simulink model "smart_sim"  (Simulink 8.0)
settings: Solver=ode45  StartTime=0.0  StopTime=256*2000  RelTol=1e-3
libraries: xbsIndex_r4 x75, simulink x1, xps_library x1
settings Model: Creator=kids  LastModifiedBy=kids

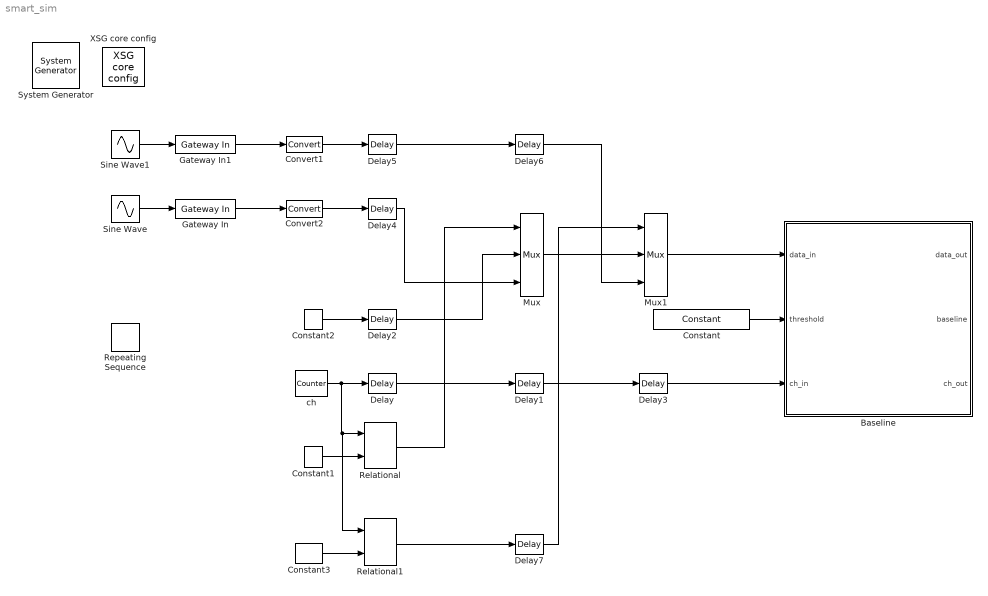
== system smart_sim ==
  " System Generator" : xbsIndex_r4/ System Generator  Tag=genX  xilinxfamily=virtex5  part=xc5vsx95t  speed=-1  package=ff1136  synthesis_tool=XST  clock_wrapper=Clock Enables  directory=./chan_dead_v1/sysgen  proj_type=Project Navigator  Synth_file=XST Defaults  Impl_file=ISE Defaults  testbench=off  simulink_period=1  sysclk_period=3.9062  dcm_input_clock_period=100  incr_netlist=off  trim_vbits=Everywhere in SubSystem  dbl_ovrd=According to Block Masks  core_generation=According to Block Masks  run_coregen=off  deprecated_control=off  eval_field=0  block_type=sysgen
      settings: block_version=10.1.3
  Baseline : Subsystem  mask{logChannels=8, logPtsInAvg=10, logSamplePeriod=1}
      mask prompts: logChannels "number of channels 2^M"; logPtsInAvg "number of samples per average 2^N"; logSamplePeriod "sampling period 2^P"
  Constant : xbsIndex_r4/Constant  const=-.1  gui_display_data_type=Fixed-point  arith_type=Signed (2's comp)  n_bits=16  bin_pt=13  preci_type=Single  exp_width=8  frac_width=24  explicit_period=off  period=1  equ=P=C  opselect=C  inp2=PCIN>>17  opr=+  inp1=P  carry=CIN  dbl_ovrd=off  block_type=constant
  Constant1 : xbsIndex_r4/Constant  const=1  gui_display_data_type=Fixed-point  arith_type=Signed (2's comp)  n_bits=4  bin_pt=0  preci_type=Single  exp_width=8  frac_width=24  explicit_period=off  period=1  equ=P=C  opselect=C  inp2=PCIN>>17  opr=+  inp1=P  carry=CIN  dbl_ovrd=off  block_type=constant
  Constant2 : xbsIndex_r4/Constant  const=0  gui_display_data_type=Fixed-point  arith_type=Signed (2's comp)  n_bits=16  bin_pt=13  preci_type=Single  exp_width=8  frac_width=24  explicit_period=on  period=1  equ=P=C  opselect=C  inp2=PCIN>>17  opr=+  inp1=P  carry=CIN  dbl_ovrd=off  block_type=constant
  Constant3 : xbsIndex_r4/Constant  const=10  gui_display_data_type=Fixed-point  arith_type=Unsigned  n_bits=4  bin_pt=0  preci_type=Single  exp_width=8  frac_width=24  explicit_period=off  period=1  equ=P=C  opselect=C  inp2=PCIN>>17  opr=+  inp1=P  carry=CIN  dbl_ovrd=off  block_type=constant
  Convert1 : xbsIndex_r4/Convert  gui_display_data_type=Fixed-point  arith_type="Signed  (2's comp)"  n_bits=16  bin_pt=13  float_type=Single  exp_bits=8  fraction_bits=24  quantization=Truncate  overflow=Wrap  en=off  latency=0  dbl_ovrd=off  pipeline=off  block_type=convert
      settings: block_version=11.4
  Convert2 : xbsIndex_r4/Convert  gui_display_data_type=Fixed-point  arith_type="Signed  (2's comp)"  n_bits=16  bin_pt=13  float_type=Single  exp_bits=8  fraction_bits=24  quantization=Truncate  overflow=Wrap  en=off  latency=0  dbl_ovrd=off  pipeline=off  block_type=convert
      settings: block_version=11.4
  Delay{,1..7} (8 alike) : xbsIndex_r4/Delay  rst=off  infoeditControl=Selection of Reset will increase slice count due to use of real FFs and instead of SRLs  en=off  latency=1  dbl_ovrd=off  reg_retiming=off  block_type=delay
  Gateway In : xbsIndex_r4/Gateway In  gui_display_data_type=Fixed-point  arith_type="Signed  (2's comp)"  n_bits=16  bin_pt=13  preci_type=Single  exp_width=8  frac_width=24  quantization="Round  (unbiased: +/- Inf)"  overflow=Saturate  period=1  dbl_ovrd=off  timing_constraint=None  locs_specified=off  LOCs={}  UseAsADC=off  ADCChannel='1'  inherit_from_input=off  hdl_port=on  block_type=gatewayin
  Gateway In1 : xbsIndex_r4/Gateway In  gui_display_data_type=Fixed-point  arith_type="Signed  (2's comp)"  n_bits=16  bin_pt=13  preci_type=Single  exp_width=8  frac_width=24  quantization="Round  (unbiased: +/- Inf)"  overflow=Saturate  period=1  dbl_ovrd=off  timing_constraint=None  locs_specified=off  LOCs={}  UseAsADC=off  ADCChannel='1'  inherit_from_input=off  hdl_port=on  block_type=gatewayin
  Mux : xbsIndex_r4/Mux  inputs=2  en=off  latency=1  precision=Full  arith_type=Unsigned  n_bits=16  bin_pt=14  quantization=Truncate  overflow=Wrap  dbl_ovrd=off  block_type=mux
  Mux1 : xbsIndex_r4/Mux  inputs=2  en=off  latency=1  precision=Full  arith_type=Unsigned  n_bits=16  bin_pt=14  quantization=Truncate  overflow=Wrap  dbl_ovrd=off  block_type=mux
  Relational : xbsIndex_r4/Relational  mode=a=b  en=off  latency=1  dbl_ovrd=off  block_type=relational
  Relational1 : xbsIndex_r4/Relational  mode=a=b  en=off  latency=1  dbl_ovrd=off  block_type=relational
  Repeating Sequence : simulink/Sources/Repeating Sequence  rep_seq_t=[0 16 16+1 2*16]  rep_seq_y=[1 1 2 2]
  Sine Wave : Sin  SineType=Sample based  Amplitude=.25  Bias=.75  Frequency=100  Samples=50*256  SampleTime=1
  Sine Wave1 : Sin  SineType=Sample based  Amplitude=.5  Bias=1.2  Frequency=100  Samples=20*256  SampleTime=1
  XSG core config : xps_library/XSG core config  Tag=xps:xsg  hw_sys=ROACH:sx95t  clk_src=adc1_clk  ROACH_clk_src=adc1_clk  ROACH2_clk_src=adc0_clk  clk_rate=256  sample_period=1  synthesis_tool=XST
  ch : xbsIndex_r4/Counter  cnt_type=Free Running  cnt_to=4  operation=Up  start_count=0  cnt_by_val=1  arith_type=Unsigned  n_bits=8  bin_pt=0  load_pin=off  rst=off  en=off  explicit_period=on  period=1  dbl_ovrd=off  use_behavioral_HDL=off  implementation=Fabric  block_type=counter
  wires:
  ch/1 -> Relational1/1, Relational/1, Delay/1
  Constant/1 -> Baseline/2(threshold)
  Constant1/1 -> Relational/2
  Constant2/1 -> Delay2/1
  Delay/1 -> Delay1/1
  Delay1/1 -> Delay3/1
  Delay2/1 -> Mux/2
  Convert2/1 -> Delay4/1
  Gateway In/1 -> Convert2/1
  Sine Wave/1 -> Gateway In/1
  Gateway In1/1 -> Convert1/1
  Sine Wave1/1 -> Gateway In1/1
  Constant3/1 -> Relational1/2
  Relational/1 -> Mux/1
  Mux/1 -> Mux1/2
  Relational1/1 -> Delay7/1
  Convert1/1 -> Delay5/1
  Mux1/1 -> Baseline/1(data_in)
  Delay3/1 -> Baseline/3(ch_in)
  Delay4/1 -> Mux/3
  Delay5/1 -> Delay6/1
  Delay6/1 -> Mux1/3
  Delay7/1 -> Mux1/1

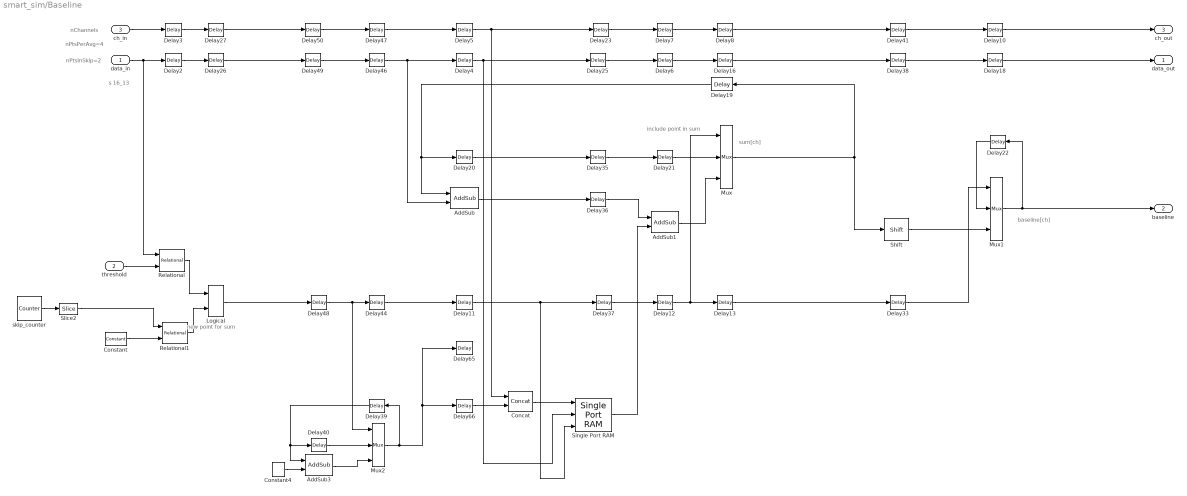
== system smart_sim/Baseline ==
  note: sum[ch]
  note: baseline[ch]
  note: nPtsInSkip=2
  note: nPtsPerAvg=4
  note: new point
      | for sum
  note: nChannels
  note: include point in sum
  note: s 16_13
  data_in : Inport
  threshold : Inport  Port=2
  ch_in : Inport  Port=3
  AddSub : xbsIndex_r4/AddSub  mode=Addition  use_carryin=off  use_carryout=off  en=off  latency=3  precision=User Defined  arith_type=Unsigned  n_bits=16+logPtsInAvg  bin_pt=13  quantization=Truncate  overflow=Wrap  dbl_ovrd=off  use_behavioral_HDL=off  hw_selection=Fabric  pipelined=off  block_type=addsub
  AddSub1 : xbsIndex_r4/AddSub  mode=Subtraction  use_carryin=off  use_carryout=off  en=off  latency=3  precision=Full  arith_type=Unsigned  n_bits=16  bin_pt=14  quantization=Truncate  overflow=Wrap  dbl_ovrd=off  use_behavioral_HDL=off  hw_selection=Fabric  pipelined=off  block_type=addsub
  AddSub3 : xbsIndex_r4/AddSub  mode=Addition  use_carryin=off  use_carryout=off  en=off  latency=3  precision=User Defined  arith_type=Unsigned  n_bits=logPtsInAvg  bin_pt=0  quantization=Truncate  overflow=Wrap  dbl_ovrd=off  use_behavioral_HDL=off  hw_selection=Fabric  pipelined=off  block_type=addsub
  Concat : xbsIndex_r4/Concat  num_inputs=2  dbl_ovrd=off  block_type=concat
  Constant : xbsIndex_r4/Constant  const=1  gui_display_data_type=Fixed-point  arith_type=Signed (2's comp)  n_bits=2  bin_pt=0  preci_type=Single  exp_width=8  frac_width=24  explicit_period=off  period=1  equ=P=C  opselect=C  inp2=PCIN>>17  opr=+  inp1=P  carry=CIN  dbl_ovrd=off  block_type=constant
  Constant4 : xbsIndex_r4/Constant  const=1  gui_display_data_type=Fixed-point  arith_type=Unsigned  n_bits=logPtsInAvg  bin_pt=0  preci_type=Single  exp_width=8  frac_width=24  explicit_period=off  period=1  equ=P=C  opselect=C  inp2=PCIN>>17  opr=+  inp1=P  carry=CIN  dbl_ovrd=off  block_type=constant
  Delay{2..3,8,10,13,16,18,23,25..27,33,35..38,41,44,46..47} (20 alike) : xbsIndex_r4/Delay  rst=off  infoeditControl=Selection of Reset will increase slice count due to use of real FFs and instead of SRLs  en=off  latency=1  dbl_ovrd=off  reg_retiming=off  block_type=delay
  Delay{4..7,11..12,20..21,40,48..50,65..66} (14 alike) : xbsIndex_r4/Delay  rst=off  infoeditControl=Selection of Reset will increase slice count due to use of real FFs and instead of SRLs  en=off  latency=3  dbl_ovrd=off  reg_retiming=off  block_type=delay
  Delay19 : xbsIndex_r4/Delay  rst=off  infoeditControl=Selection of Reset will increase slice count due to use of real FFs and instead of SRLs  en=off  latency=2^logChannels-8  dbl_ovrd=off  reg_retiming=off  block_type=delay
  Delay22 : xbsIndex_r4/Delay  rst=off  infoeditControl=Selection of Reset will increase slice count due to use of real FFs and instead of SRLs  en=off  latency=2^logChannels-1  dbl_ovrd=off  reg_retiming=off  block_type=delay
  Delay39 : xbsIndex_r4/Delay  rst=off  infoeditControl=Selection of Reset will increase slice count due to use of real FFs and instead of SRLs  en=off  latency=2^logChannels-4  dbl_ovrd=off  reg_retiming=off  block_type=delay
  Logical : xbsIndex_r4/Logical  logical_function=AND  inputs=2  en=off  latency=1  precision=Full  arith_type=Unsigned  n_bits=16  bin_pt=0  align_bp=on  dbl_ovrd=off  block_type=logical
  Mux : xbsIndex_r4/Mux  inputs=2  en=off  latency=1  precision=Full  arith_type=Unsigned  n_bits=16  bin_pt=14  quantization=Truncate  overflow=Wrap  dbl_ovrd=off  block_type=mux
  Mux1 : xbsIndex_r4/Mux  inputs=2  en=off  latency=1  precision=Full  arith_type=Unsigned  n_bits=16  bin_pt=14  quantization=Truncate  overflow=Wrap  dbl_ovrd=off  block_type=mux
  Mux2 : xbsIndex_r4/Mux  inputs=2  en=off  latency=1  precision=Full  arith_type=Unsigned  n_bits=16  bin_pt=14  quantization=Truncate  overflow=Wrap  dbl_ovrd=off  block_type=mux
  Relational : xbsIndex_r4/Relational  mode=a>b  en=off  latency=1  dbl_ovrd=off  block_type=relational
  Relational1 : xbsIndex_r4/Relational  mode=a=b  en=off  latency=1  dbl_ovrd=off  block_type=relational
  Shift : xbsIndex_r4/Shift  shift_dir=Right  shift_bits=logPtsInAvg  en=off  latency=1  precision=User Defined  arith_type="Signed  (2's comp)"  n_bits=16  bin_pt=13  quantization=Truncate  overflow=Wrap  dbl_ovrd=off  block_type=shift
  Single Port RAM : xbsIndex_r4/Single Port RAM  depth=2^logChannels*2^logPtsInAvg  initVector=0  distributed_mem=Block RAM  write_mode=Read Before Write  rst=off  init_reg=0  en=off  latency=1  dbl_ovrd=off  optimize=Area  block_type=spram
  Slice2 : xbsIndex_r4/Slice  nbits=logSamplePeriod  boolean_output=off  mode=Upper Bit Location + Width  bit1=0  base1=MSB of Input  bit0=0  base0=LSB of Input  dbl_ovrd=off  block_type=slice
      settings: block_version=10.1.3
  skip_counter : xbsIndex_r4/Counter  cnt_type=Free Running  cnt_to=Inf  operation=Up  start_count=0  cnt_by_val=1  arith_type=Unsigned  n_bits=logSamplePeriod+logChannels  bin_pt=0  load_pin=off  rst=off  en=off  explicit_period=on  period=1  dbl_ovrd=off  use_behavioral_HDL=off  implementation=Fabric  block_type=counter
  data_out : Outport
  baseline : Outport  Port=2
  ch_out : Outport  Port=3
  wires:
  data_in/1 -> Delay2/1, Relational/1
  threshold/1 -> Relational/2
  Constant/1 -> Relational1/2
  skip_counter/1 -> Slice2/1
  Relational/1 -> Logical/1
  AddSub/1 -> Delay36/1
  ch_in/1 -> Delay3/1
  Shift/1 -> Mux1/3
  Delay2/1 -> Delay26/1
  Delay3/1 -> Delay27/1
  Mux/1 -> Delay19/1, Shift/1
  Delay5/1 -> Concat/1, Delay23/1
  Delay6/1 -> Delay16/1
  Delay7/1 -> Delay8/1
  Delay8/1 -> Delay41/1
  Delay11/1 -> Single Port RAM/3, Delay37/1
  Delay12/1 -> Delay13/1, Mux/1
  Delay13/1 -> Delay33/1
  Delay16/1 -> Delay38/1
  Delay19/1 -> AddSub/1, Delay20/1
  Delay20/1 -> Delay35/1
  Delay21/1 -> Mux/2
  Delay22/1 -> Mux1/2
  Delay27/1 -> Delay50/1
  Delay18/1 -> data_out/1
  Mux1/1 -> baseline/1, Delay22/1
  Delay26/1 -> Delay49/1
  Delay23/1 -> Delay7/1
  Delay25/1 -> Delay6/1
  Delay35/1 -> Delay21/1
  Delay36/1 -> AddSub1/1
  Delay37/1 -> Delay12/1
  Mux2/1 -> Delay39/1, Delay65/1, Delay66/1
  Delay44/1 -> Delay11/1
  Delay46/1 -> AddSub/2, Delay4/1
  Delay47/1 -> Delay5/1
  Single Port RAM/1 -> AddSub1/2
  Concat/1 -> Single Port RAM/1
  Delay49/1 -> Delay46/1
  Delay39/1 -> Delay40/1, AddSub3/1
  AddSub3/1 -> Mux2/3
  Constant4/1 -> AddSub3/2
  Delay40/1 -> Mux2/2
  Delay48/1 -> Mux2/1, Delay44/1
  Delay50/1 -> Delay47/1
  AddSub1/1 -> Mux/3
  Slice2/1 -> Relational1/1
  Logical/1 -> Delay48/1
  Delay4/1 -> Delay25/1, Single Port RAM/2
  Delay33/1 -> Mux1/1
  Delay38/1 -> Delay18/1
  Delay41/1 -> Delay10/1
  Relational1/1 -> Logical/2
  Delay66/1 -> Concat/2
  Delay10/1 -> ch_out/1
